simulink model "TankAndControllerWithStateflow"  (Simulink 8.1)
settings: Solver=ode23tb  StartTime=0.0  StopTime=30  RelTol=1e-3
settings Model: Creator=root  LastModifiedBy=root
settings DataIOCC: SignalLoggingSaveFormat=Dataset
settings OptimizationCC: ExpressionDepthLimit=128
settings DebuggingCC: FcnCallInpInsideContextMsg=EnableAllAsError
settings GRTTargetCC: CombineOutputUpdateFcns=on  GRTInterface=off

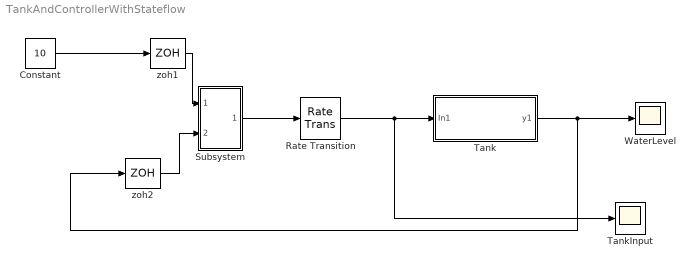
== system TankAndControllerWithStateflow ==
  Constant : Constant  Value=10
  Rate Transition : RateTransition
  Subsystem : Subsystem
  Tank : Subsystem
  TankInput : Scope
  WaterLevel : Scope
      settings: YMin=0  YMax=14
  "zoh1 " : ZeroOrderHold  SampleTime=0.01
  "zoh2 " : ZeroOrderHold  SampleTime=0.01
  wires:
  Constant/1 -> "zoh1 "/1
  Tank/1(y1) -> "zoh2 "/1, WaterLevel/1
  Subsystem/1(Out1) -> Rate Transition/1
  "zoh1 "/1 -> Subsystem/1(In1)
  "zoh2 "/1 -> Subsystem/2(In2)
  Rate Transition/1 -> TankInput/1, Tank/1(In1)

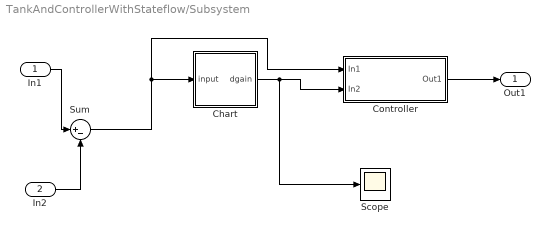
== system TankAndControllerWithStateflow/Subsystem ==
  In1 : Inport
  In2 : Inport  Port=2
  Chart : Stateflow chart  TreatAsAtomicUnit=on
  Controller : Subsystem
  Scope : Scope
      settings: SaveName=ScopeData2
  Sum : Sum  Inputs=|+-
  Out1 : Outport
  wires:
  Controller/1(Out1) -> Out1/1
  In1/1 -> Sum/1
  Chart/1(dgain) -> Scope/1, Controller/2(In2)
  Sum/1 -> Controller/1(In1), Chart/1(input)
  In2/1 -> Sum/2

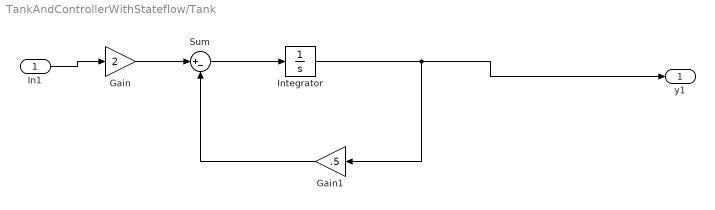
== system TankAndControllerWithStateflow/Tank ==
  In1 : Inport
  Gain : Gain  Gain=2
  Gain1 : Gain  Gain=.5
  Integrator : Integrator
  Sum : Sum  Inputs=|+-
  y1 : Outport
  wires:
  In1/1 -> Gain/1
  Gain/1 -> Sum/1
  Sum/1 -> Integrator/1
  Integrator/1 -> Gain1/1, y1/1
  Gain1/1 -> Sum/2

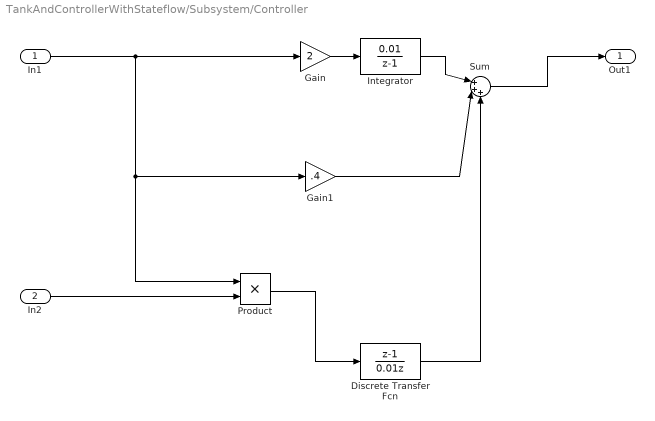
== system TankAndControllerWithStateflow/Subsystem/Controller ==
  In1 : Inport
  In2 : Inport  Port=2
  Discrete Transfer Fcn : DiscreteTransferFcn  Numerator=[1 -1]  Denominator=[0.01 0]  SampleTime=0.01
  Gain : Gain  Gain=2
  Gain1 : Gain  Gain=.4
  Integrator : DiscreteTransferFcn  Numerator=[0.01]  Denominator=[1 -1]  SampleTime=0.01
  Product : Product
  Sum : Sum  Inputs=|+++
  Out1 : Outport
  wires:
  In1/1 -> Product/1, Gain1/1, Gain/1
  Gain/1 -> Integrator/1
  Integrator/1 -> Sum/1
  Gain1/1 -> Sum/2
  Sum/1 -> Out1/1
  Discrete Transfer Fcn/1 -> Sum/3
  In2/1 -> Product/2
  Product/1 -> Discrete Transfer Fcn/1

== stateflow chart Subsystem/Chart ==
  state GainOn
    entry: dgain = 0.2
  state GainOff
    entry: dgain = 0
  (default) -> GainOn : {dgain = 0.2}
  GainOff -> GainOn : [input > 6]
  GainOn -> GainOff : [input < 2]
  data: input input double; dgain output double
